simulink model "Ch2"  (R2018b)
settings: Solver=VariableStepAuto  StartTime=0.0  StopTime=1.0  RelTol=1e-3
settings Model: Creator=Mahdi  LastModifiedBy=Mahdi

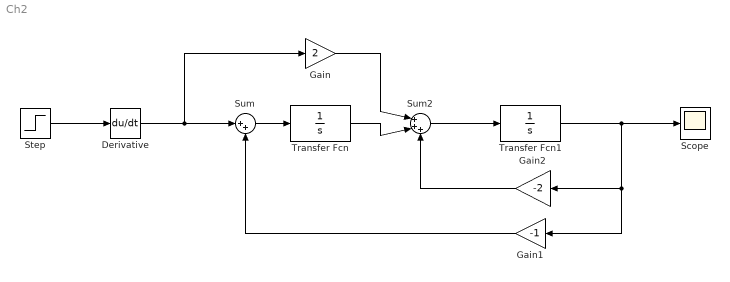
== system Ch2 ==
  Derivative : Derivative
  Gain : Gain  Gain=2
  Gain1 : Gain  Gain=-1
  Gain2 : Gain  Gain=-2
  Scope : Scope
  Step : Step  Time=0.001  SampleTime=0
  Sum : Sum  Inputs=|++
  Sum2 : Sum  Inputs=|+++
  Transfer Fcn : TransferFcn  Denominator=[1 0]
  Transfer Fcn1 : TransferFcn  Denominator=[1 0]
  wires:
  Sum/1 -> Transfer Fcn/1
  Gain1/1 -> Sum/2
  Transfer Fcn1/1 -> Gain1/1, Gain2/1, Scope/1
  Step/1 -> Derivative/1
  Derivative/1 -> Gain/1, Sum/1
  Transfer Fcn/1 -> Sum2/2
  Gain/1 -> Sum2/1
  Gain2/1 -> Sum2/3
  Sum2/1 -> Transfer Fcn1/1
